simulink model "Simulink_total_missing_gen_and_coils"  (R2024a)
settings: Solver=VariableStepAuto  StartTime=0.0  StopTime=10.0  RelTol=1e-3
libraries: spsDiodeLib x5, spsMosfetLib x5, spsSeriesRLCBranchLib x4, spsVoltageMeasurementLib x3, spsCurrentMeasurementLib x2, spsDCVoltageSourceLib x1, spspowerguiLib x1
settings Model: Creator=20212044  LastModifiedBy=20212044

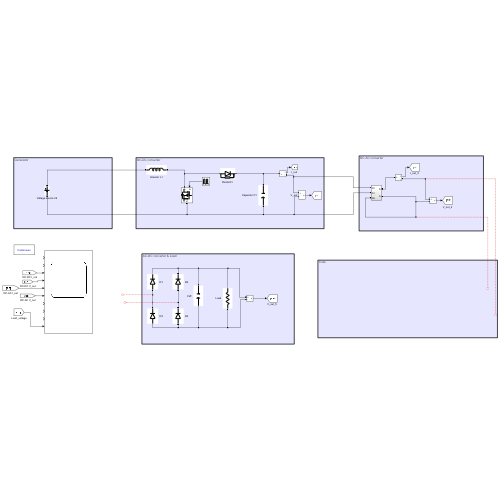
[thumbnail: Simulink's stored preview of the top-level diagram]
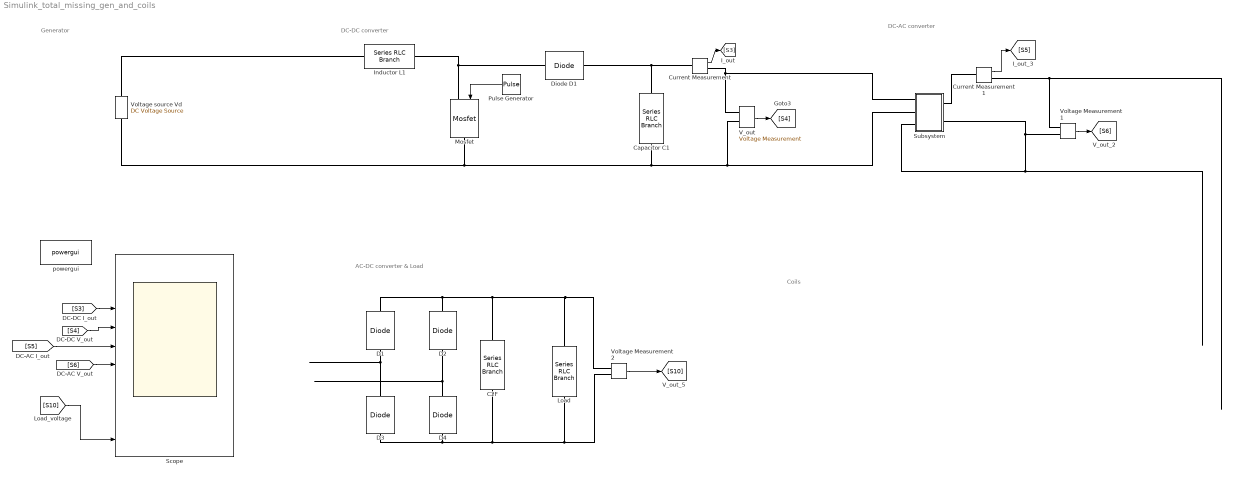
== system Simulink_total_missing_gen_and_coils ==
  note: Generator
  note: AC-DC converter & Load
  note: Coils
  note: DC-AC converter
  note: DC-DC converter
  C2F : spsSeriesRLCBranchLib/Series RLC Branch  LConnTagsString=__new0  RConnTagsString=__new0  BranchType=C  Resistance=1e-6  Inductance=1e-3  SetiL0=off  InitialCurrent=0  Capacitance=300e-6  Setx0=off  InitialVoltage=0  Measurements=Branch voltage
  Capacitor C1 : spsSeriesRLCBranchLib/Series RLC Branch  LConnTagsString=__new0  RConnTagsString=__new0  BranchType=C  Resistance=1  Inductance=1e-3  SetiL0=off  InitialCurrent=0  Capacitance=220e-6  Setx0=off  InitialVoltage=0  Measurements=None
  Current Measurement : spsCurrentMeasurementLib/Current Measurement  PhasorSimulation=off  OutputType=Complex  PSBequivalent=0
  Current Measurement1 : spsCurrentMeasurementLib/Current Measurement  PhasorSimulation=off  OutputType=Complex  PSBequivalent=0
  D{1..4} (4 alike) : spsDiodeLib/Diode  Ron=0.001  Lon=0  Vf=0.8  IC=0  UseSnubber=0  Rs=0  Cs=0  Measurements=off
  Diode D1 : spsDiodeLib/Diode  Ron=0.001  Lon=0  Vf=0.8  IC=0  UseSnubber=0  Rs=500  Cs=250e-9  Measurements=off
  Inductor L1 : spsSeriesRLCBranchLib/Series RLC Branch  LConnTagsString=__new0  RConnTagsString=__new0  BranchType=L  Resistance=1  Inductance=50e-6  SetiL0=off  InitialCurrent=0  Capacitance=1e-6  Setx0=off  InitialVoltage=0  Measurements=None
  Load : spsSeriesRLCBranchLib/Series RLC Branch  LConnTagsString=__new0  RConnTagsString=__new0  BranchType=R  Resistance=10  Inductance=1e-3  SetiL0=off  InitialCurrent=0  Capacitance=1e-6  Setx0=off  InitialVoltage=0  Measurements=None
  Mosfet : spsMosfetLib/Mosfet  Ron=0.1  Lon=0  Rd=0.01  Vfd=0  IC=0  Rs=1e5  Cs=inf  Measurements=off
  Pulse Generator : DiscretePulseGenerator  PulseType=Time based  Period=1/20000  PulseWidth=20
  Scope : Scope  NumInputPorts=10
  Subsystem : Subsystem
  V_out : spsVoltageMeasurementLib/Voltage Measurement  PhasorSimulation=off  OutputType=Complex  PSBequivalent=0
  Voltage Measurement1 : spsVoltageMeasurementLib/Voltage Measurement  PhasorSimulation=off  OutputType=Complex  PSBequivalent=0
  Voltage Measurement2 : spsVoltageMeasurementLib/Voltage Measurement  PhasorSimulation=off  OutputType=Complex  PSBequivalent=0
  Voltage source Vd : spsDCVoltageSourceLib/DC Voltage Source  Amplitude=30  Measurements=None
  powergui : spspowerguiLib/powergui  Priority=1  SimulationMode=Continuous  SampleTime=50e-6  frequency=60  Iterations=50  frequencyindice=0  Pbase=100e6  ErrMax=1e-4  UnitsV=kV  UnitsW=MW  buscounter=0  FunctionMessages=off  echomessages=off  EnableUseOfTLC=off  CurrentSourceSwitches=off  DisableSnubberDevices=off  DisableRonSwitches=off  DisableVfSwitches=off  DisplayEquations=off  AutomaticDiscreteSolvers=off  SolverType=Tustin/Backward Euler (TBE)  Interpol=off  ExternalGateDelay=off  methode=off  Ts=100  x0status=blocks  SPID=on  SwTol=0  HookPort=off  NonlinearTolerance=1e-4  nMaxIteration=100  ContinueOnMaxIteration=off  RestoreLinks=warning  ResistiveCurrentMeasurement=off  Frange=[0:2:500]  Ylog=off  Xlog=on  ShowGrid=off  save=off  variable=ZData  structure=0  ZoomFFT=off  StartTime=0.0  cycles=1  DisplayStyle=1  fundamental=60  FreqAxis=off  MaxFrequency=1000  frequencyindicesteady=1  RmsSteady=1  display=off
  wires:
  [S3] -> Scope/3
  Pulse Generator/1 -> Mosfet/1
  V_out/1 -> [S4]
  [S4] -> Scope/4
  Current Measurement/1 -> [S3]
  Voltage Measurement2/1 -> [S10]
  [S10] -> Scope/10
  Current Measurement1/1 -> [S5]
  Voltage Measurement1/1 -> [S6]
  [S6] -> Scope/6
  [S5] -> Scope/5
  connections:
  V_out/LConn2 -- Subsystem/LConn2 -- Mosfet/RConn1 -- Voltage source Vd/LConn1 -- Capacitor C1/RConn1
  Diode D1/LConn1 -- Mosfet/LConn1 -- Inductor L1/RConn1
  V_out/LConn1 -- Current Measurement/RConn1 -- Subsystem/LConn1
  Diode D1/RConn1 -- Capacitor C1/LConn1 -- Current Measurement/LConn1
  Inductor L1/LConn1 -- Voltage source Vd/RConn1
  D2/RConn1 -- C2F/LConn1 -- Load/LConn1 -- Voltage Measurement2/LConn1 -- D1/RConn1
  D3/RConn1 -- D1/LConn1
  D2/LConn1 -- D4/RConn1
  D3/LConn1 -- Load/RConn1 -- Voltage Measurement2/LConn2 -- C2F/RConn1 -- D4/LConn1
  Subsystem/LConn3 -- Voltage Measurement1/LConn2 -- Subsystem/RConn2
  Voltage Measurement1/LConn1 -- Current Measurement1/RConn1
  Current Measurement1/LConn1 -- Subsystem/RConn1

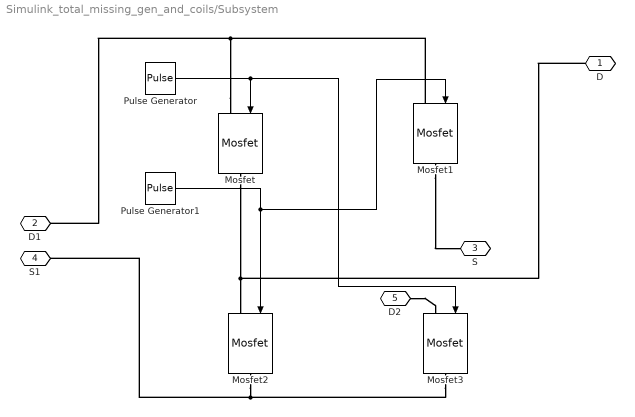
== system Simulink_total_missing_gen_and_coils/Subsystem ==
  Mosfet{,1..3} (4 alike) : spsMosfetLib/Mosfet  Ron=0.15  Lon=0  Rd=0.01  Vfd=1.0  IC=0  Rs=1e5  Cs=inf  Measurements=off
  Pulse Generator : DiscretePulseGenerator  PulseType=Time based  Period=1/80000  PulseWidth=50
  Pulse Generator1 : DiscretePulseGenerator  PulseType=Time based  Period=1/80000  PulseWidth=50  PhaseDelay=1/80000/2
  D : PMIOPort  Side=Right
  D1 : PMIOPort  Port=2  Side=Left
  S : PMIOPort  Port=3  Side=Right
  S1 : PMIOPort  Port=4  Side=Left
  D2 : PMIOPort  Port=5  Side=Left
  wires:
  Pulse Generator/1 -> Mosfet3/1, Mosfet/1
  Pulse Generator1/1 -> Mosfet1/1, Mosfet2/1
  connections:
  Mosfet/LConn1 -- D1/RConn1 -- Mosfet1/LConn1
  Mosfet2/RConn1 -- S1/RConn1 -- Mosfet3/RConn1
  Mosfet/RConn1 -- D/RConn1 -- Mosfet2/LConn1
  D2/RConn1 -- Mosfet3/LConn1
  Mosfet1/RConn1 -- S/RConn1
